simulink model "Appl_DrMotorAdjust_CtrlModel"  (R2018b)
settings: configuration reference "CodeConfig_10_ms" (kept outside this file)
undefined symbols (not defined in the file): CAL_HightMotorRunInterval_100ms, CAL_MotorDiffToStart_100ms, CAL_MotorStopTime_50ms, D_Relay_DownBackFault, D_Relay_UpFrontFault, D_ToleranceDistance, enSeatMoveCmd, FALSE, TRUE
libraries: DareLib x88, simulink x2
(part 3 of 3)

== stateflow chart Appl_DrMotorAdjust_CtrlModel/LogicCtrl/LocalAdjustCtrl/MotorAdjust/LengthMotorRun/MotorAdjust ==
  note: 此处取霍尔值越往下越大约往后越大
  state Init_Interval
    en:
    H_SeatMoveCmd = enSeatMoveCmd.EN_NULL;
    HMotorRunIntervalTime = 1;
    DownBackFlag = 0;
    UpFrontFlag = 0;
    Testvalue = 1;
    du:
    ex:
    HMotorRunIntervalTime = 0;
    Init_Interval -> (junction 11) [order 1]
    (junction 11) -> (junction 13) [order 1] : /*纵向电机调间隔时间*/
        | [HMotorRunIntervalTime < CAL_HightMotorRunInterval_100ms]
    (junction 11) -> (junction 17) [order 2]
    (junction 13) -> (junction 15) : {HMotorRunIntervalTime ++;}
    (junction 15) -> (junction 17)
    (junction 17) -> (junction 30) : {DownBackFlag = 0;
        | UpFrontFlag = 0;}
    (junction 30) -> (junction 32) [order 1] : /*纵向自动调节有效*/
        | [0 != SeatHeightPosiReq]
    (junction 32) -> (junction 43) [order 1] : /*纵向误差判断目前定义为5霍尔数值*/
        | [enSeatMoveCmd.EN_UP_FORWARD != LengthSoftStopFault ...
        | && SeatHeightPosiReq > DrAdj_InCurrentHallCnt ...
        | && D_ToleranceDistance < (SeatHeightPosiReq - DrAdj_InCurrentHallCnt)]
    (junction 30) -> (junction 39) [order 2] : { HeightAutoRunFlag = EN_SEAT_INVALID;}
    (junction 32) -> (junction 34) [order 2]
    (junction 43) -> (junction 45) : {UpFrontFlag = 1;}
    (junction 34) -> (junction 47) [order 1] : /* 不在软止点 且超误差范围 */
        | [enSeatMoveCmd.EN_DN_BACKWARD != LengthSoftStopFault ...
        | && SeatHeightPosiReq < DrAdj_InCurrentHallCnt ...
        | && D_ToleranceDistance < (DrAdj_InCurrentHallCnt - SeatHeightPosiReq)]
    (junction 34) -> (junction 52) [order 2] : /*纵向误差范围内，反馈成功*/
        | {HeightAutoRunFlag = EN_SEAT_SUCCESS;
        | H_MotorRunType = EN_AutoAdjust_FUSuccess_Stop;}
    (junction 47) -> (junction 49) : {DownBackFlag = 1;}
    (junction 52) -> (junction 39)
    (junction 49) -> (junction 52)
    (junction 45) -> (junction 49)
    (junction 39) -> (junction 57)
    (junction 57) -> (junction 134)
    (junction 134) -> (junction 135) [order 1] : /* 调用位置有变化 则先清状态 */
        | [hasChanged(SeatHeightPosiReq)]
    (junction 134) -> (junction 133) [order 2]
    (junction 135) -> (junction 126) : {HeightAutoRunFlag = EN_SEAT_INVALID;}
    (junction 126) -> (junction 133)
    (junction 133) -> (junction 128)
  state H_MotorUpFrontRun
    en:
    H_SeatMoveCmd  = EN_UP_FORWARD
    Testvalue = 2;
    (default) -> (junction 64)
    H_MotorUpFrontRun -> (junction 64) [order 1]
    (junction 64) -> (junction 67) [order 1] : /*自动调节*/
        | [EN_AutoAdjust_FU == H_MotorRunType]
    (junction 64) -> (junction 71) [order 2] : {HeightAutoRunFlag = EN_SEAT_INVALID;}
    (junction 67) -> (junction 69) : {HeightAutoRunFlag = EN_SEAT_RUNNING;}
    (junction 69) -> (junction 71)
    (junction 71) -> (junction 74)
  state H_MotorDownBackRun
    en:
    H_SeatMoveCmd  = EN_DN_BACKWARD;
    Testvalue = 3;
    (default) -> (junction 87)
    H_MotorDownBackRun -> (junction 87) [order 1]
    (junction 87) -> (junction 81) [order 1] : /*纵向自动调节*/
        | [EN_AutoAdjust_BK == H_MotorRunType]
    (junction 87) -> (junction 84) [order 2] : {HeightAutoRunFlag = EN_SEAT_INVALID;}
    (junction 81) -> (junction 77) : {HeightAutoRunFlag = EN_SEAT_RUNNING;}
    (junction 77) -> (junction 84)
    (junction 84) -> (junction 89)
  (default) -> Init_Interval
  Init_Interval -> H_MotorUpFrontRun [order 4] : /*纵向继电器下后粘连故障 == 有效 间隔时间大于100ms*/
      | [Relay_DownBackFault ==  Relay_FaultSts...
      | && CAL_HightMotorRunInterval_100ms <= HMotorRunIntervalTime ]
      | /H_MotorRunType = EN_DnBkRelayAdhesion_FU;
  Init_Interval -> H_MotorDownBackRun [order 1] : /*纵向继电器上前粘连故障 == 有效*/
      | [Relay_UpFrontFault == Relay_FaultSts ...
      | && CAL_HightMotorRunInterval_100ms <= HMotorRunIntervalTime ]
      | /H_MotorRunType = EN_DnFURelayAdhesion_BK;
  H_MotorUpFrontRun -> Init_Interval [order 3] : /*纵向继电器下后粘连故障 != 有效*/
      | [Relay_DownBackFault != Relay_FaultSts...
      | && EN_DnBkRelayAdhesion_FU == H_MotorRunType]
      | /H_MotorRunType = EN_DnBkRelayAdhesion_FU_Stop;
  H_MotorDownBackRun -> Init_Interval [order 9] : /*纵向继电器上前粘连故障 ！= 有效*/
      | [Relay_UpFrontFault != Relay_FaultSts  ...
      | && EN_DnFURelayAdhesion_BK == H_MotorRunType]
      | /H_MotorRunType = EN_DnFURelayAdhesion_BK_Stop;
  Init_Interval -> H_MotorUpFrontRun [order 3] : /*纵向手动调节*/
      | [EN_UP_FORWARD == HeightManualAdjSw ...
      | && FALSE == LengthLockFault  ...
      | && FALSE == LengthHallFault ...
      | && FALSE == TimeoutFlag ...
      | && CAL_HightMotorRunInterval_100ms <= HMotorRunIntervalTime]
      | /H_MotorRunType = EN_ManualAdjust_FU;
  Init_Interval -> H_MotorDownBackRun [order 6] : /*纵向手动调节有效*/
      | [EN_DN_BACKWARD == HeightManualAdjSw ...
      | && FALSE == LengthLockFault   ...
      | && FALSE == LengthHallFault...
      | && FALSE == TimeoutFlag ...
      | && CAL_HightMotorRunInterval_100ms <= HMotorRunIntervalTime]
      | /H_MotorRunType = EN_ManualAdjust_BK;
  H_MotorUpFrontRun -> Init_Interval [order 5] : /*纵向手动调节无效*/
      | [(EN_UP_FORWARD != HeightManualAdjSw) ...
      | && EN_ManualAdjust_FU == H_MotorRunType]
      | /H_MotorRunType = EN_ManualAdjust_FU_Stop;
  H_MotorDownBackRun -> Init_Interval [order 7] : /*纵向手动调节无效*/
      | [(EN_DN_BACKWARD != HeightManualAdjSw) ...
      | && EN_ManualAdjust_BK == H_MotorRunType]
      | /H_MotorRunType = EN_ManualAdjust_BK_Stop;
  Init_Interval -> H_MotorUpFrontRun [order 5] : /*纵向自动调节有效且不在误差范围内*/
      | [0 != SeatHeightPosiReq ...
      | && FALSE == LengthLockFault ...
      | && HeightAutoRunFlag == EN_SEAT_INVALID ...
      | && UpFrontFlag == 1 ...
      | && CAL_HightMotorRunInterval_100ms <= HMotorRunIntervalTime]
      | /H_MotorRunType = EN_AutoAdjust_FU;
  Init_Interval -> H_MotorDownBackRun [order 2] : /*纵向自动调节有效且不在误差范围内*/
      | [0 != SeatHeightPosiReq ...
      | && FALSE == LengthLockFault ...
      | && HeightAutoRunFlag == EN_SEAT_INVALID ...
      | && DownBackFlag == 1 ...
      | && CAL_HightMotorRunInterval_100ms <= HMotorRunIntervalTime]
      | /H_MotorRunType = EN_AutoAdjust_BK;
  H_MotorDownBackRun -> Init_Interval [order 3] : /*纵向自动调节无效 设置电机运行类型BK停止 自动运行标志位失败*/
      | [0 == SeatHeightPosiReq ...
      | && EN_AutoAdjust_BK == H_MotorRunType]
      | /H_MotorRunType = EN_AutoAdjust_BK_Stop;
      | HeightAutoRunFlag =EN_SEAT_FAIL;
  H_MotorUpFrontRun -> Init_Interval [order 6] : /*纵向自动调节无效 设置电机运行类型FU停止 自动运行标志位失败*/
      | [0 == SeatHeightPosiReq ...
      | && EN_AutoAdjust_FU == H_MotorRunType]
      | /H_MotorRunType = EN_AutoAdjust_FU_Stop;
      | HeightAutoRunFlag =EN_SEAT_FAIL
  H_MotorUpFrontRun -> Init_Interval [order 7] : /*纵向自动调节成功 设置电机运行类型FU成功停止 自动运行标志位成功*/
      | [EN_AutoAdjust_FU == H_MotorRunType ...
      | && D_ToleranceDistance >= abs(SeatHeightPosiReq -  DrAdj_InCurrentHallCnt)]
      | /HeightAutoRunFlag = EN_SEAT_SUCCESS;
      | H_MotorRunType = EN_AutoAdjust_FUSuccess_Stop;
  H_MotorDownBackRun -> Init_Interval [order 4] : /*自动调节成功 设置电机运行类型成功停止 自动运行标志位成功*/
      | [EN_AutoAdjust_BK == H_MotorRunType ...
      | && D_ToleranceDistance >= abs(DrAdj_InCurrentHallCnt  - SeatHeightPosiReq)]
      | /HeightAutoRunFlag = EN_SEAT_SUCCESS;
      | H_MotorRunType = EN_AutoAdjust_BKSuccess_Stop;
  H_MotorUpFrontRun -> Init_Interval [order 9] : /*纵向超时停止-非继电器粘连的驱动*/
      | [TRUE == TimeoutFlag ...
      | && Relay_DownBackFault !=  Relay_FaultSts]
      | /H_MotorRunType = EN_AutoAdjust_FUSuccess_Stop;
      | HeightAutoRunFlag =EN_SEAT_FAIL;
  H_MotorDownBackRun -> Init_Interval [order 8] : /*纵向超时停止-非继电器粘连的驱动*/
      | [TRUE == TimeoutFlag ...
      | && Relay_UpFrontFault != Relay_FaultSts]
      | /H_MotorRunType = EN_AutoAdjust_BKSuccess_Stop;
      | HeightAutoRunFlag =EN_SEAT_FAIL;
  H_MotorUpFrontRun -> Init_Interval [order 4] : /* 纵向向前到达止点，存在堵转故障，反馈成功 */
      | [/*FALSE == Relay_FaultSts &&*/ TRUE == LengthLockFault]
      | /H_MotorRunType = enSeatHightMotorRunsts.EN_UpFn_Lock_Stop;
      | HeightAutoRunFlag =EN_SEAT_SUCCESS;
  H_MotorDownBackRun -> Init_Interval [order 6] : /* 纵向向后到达止点，存在堵转故障，反馈成功 */
      | [/*FALSE == Relay_FaultSts &&*/ TRUE == LengthLockFault]/
      | H_MotorRunType = enSeatHightMotorRunsts.EN_DnBa_Lock_Stop;
      | HeightAutoRunFlag =EN_SEAT_SUCCESS;
  H_MotorUpFrontRun -> Init_Interval [order 10] : /* 纵向存在霍尔故障 */
      | [/*FALSE == Relay_FaultSts && */TRUE == LengthHallFault]
      | /H_MotorRunType = enSeatHightMotorRunsts.EN_UpFn_Hall_Stop;
      | HeightAutoRunFlag =EN_SEAT_FAIL;
  H_MotorDownBackRun -> Init_Interval [order 10] : /* 存在霍尔故障 */
      | [/*FALSE == Relay_FaultSts &&*/ TRUE == LengthHallFault]
      | /H_MotorRunType = enSeatHightMotorRunsts.EN_DnBa_Hall_Stop;
      | HeightAutoRunFlag =EN_SEAT_FAIL;
  H_MotorUpFrontRun -> Init_Interval [order 11] : /* 纵向存在MOS故障 */
      | [enMosErrSts.enNULL != MosErrSts]
      | /H_MotorRunType = enSeatHightMotorRunsts.EN_DnBa_MovTypeChange + MosErrSts;
      | HeightAutoRunFlag =EN_SEAT_FAIL;
  H_MotorDownBackRun -> Init_Interval [order 11] : /* 存在MOS故障 */
      | [enMosErrSts.enNULL != MosErrSts]
      | /H_MotorRunType = enSeatHightMotorRunsts.EN_DnBa_MovTypeChange + MosErrSts;
      | HeightAutoRunFlag =EN_SEAT_FAIL;
  H_MotorDownBackRun -> Init_Interval [order 2] : /*自动调节-到达软止点停止 成功 */
      |  [EN_AutoAdjust_BK == H_MotorRunType ...
      | && enSeatMoveCmd.EN_DN_BACKWARD == LengthSoftStopFault]
      | /HeightAutoRunFlag = EN_SEAT_SUCCESS;
      | H_MotorRunType = EN_AutoAdjust_BKSuccess_Stop;
  H_MotorUpFrontRun -> Init_Interval [order 1] : /*自动调节-到达软止点停止 成功 */
      |  [EN_AutoAdjust_FU == H_MotorRunType ...
      | && enSeatMoveCmd.EN_UP_FORWARD == LengthSoftStopFault]
      | /HeightAutoRunFlag = EN_SEAT_SUCCESS;
      | H_MotorRunType = EN_AutoAdjust_FUSuccess_Stop;
  H_MotorDownBackRun -> Init_Interval [order 1] : /*纵向控制类型改变
      | 优先级需要设定为1*/
      | [hasChanged(MotorActType)...
      |  && enSeatMotorRunTye.EN_NULL != MotorActType]
      | /HeightAutoRunFlag = EN_SEAT_INVALID;
      | H_MotorRunType = EN_DnBa_MovTypeChange;
  H_MotorUpFrontRun -> Init_Interval [order 2] : /*纵向控制类型改变
      | 不能返回运动成功优先级需要设定为1*/
      | [hasChanged(MotorActType)...
      |  && enSeatMotorRunTye.EN_NULL != MotorActType]
      | /HeightAutoRunFlag = EN_SEAT_INVALID;
      | H_MotorRunType = EN_UpFn_MovTypeChange
  H_MotorDownBackRun -> Init_Interval [order 5] : /* 不在软止点 且超过误差范围，需要向前驱动 */
      | [0 != SeatHeightPosiReq ...
      | && SeatHeightPosiReq > DrAdj_InCurrentHallCnt]
      | /HeightAutoRunFlag = EN_SEAT_INVALID;
      | H_MotorRunType = EN_AutoAdjust_BK_Stop;
  H_MotorUpFrontRun -> Init_Interval [order 8] : /* 不在软止点 且超过误差范围，需要向后驱动 */
      | [0 != SeatHeightPosiReq ...
      | && SeatHeightPosiReq < DrAdj_InCurrentHallCnt]
      | /HeightAutoRunFlag = EN_SEAT_INVALID;
      | H_MotorRunType = EN_AutoAdjust_FU_Stop;
  data: TimeoutFlag input; DrAdj_InCurrentHallCnt input; Relay_FaultSts input; SeatHeightPosiReq input; HeightManualAdjSw input; H_SeatMoveCmd output Enum: enSeatMoveCmd; H_MotorRunType output Enum: enSeatHightMotorRunsts; CAL_HightMotorRunInterval_100ms input; DownBackFlag local uint8; UpFrontFlag local uint8; HeightAutoRunFlag output Enum: enSeatAutoRunSts; TRUE input; HMotorRunIntervalTime local uint8 =10; Relay_DownBackFault input; Relay_UpFrontFault input; LengthHallFault input; LengthLockFault input; FALSE parameter; LengthSoftStopFault input; MotorActType input; D_ToleranceDistance input; Testvalue output uint8; MosErrSts input Enum: enMosErrSts

== stateflow chart Appl_DrMotorAdjust_CtrlModel/LogicCtrl/LocalAdjustCtrl/MotorAdjust/BackMotorRun/MotorAdjust ==
  note: 此处取霍尔值越往下越大约往后越大
  state Init_Interval
    en:
    H_SeatMoveCmd = enSeatMoveCmd.EN_NULL;
    HMotorRunIntervalTime = 1;
    DownBackFlag = 0;
    UpFrontFlag = 0;
    Testvalue = 1;
    du:
    ex:
    HMotorRunIntervalTime = 0;
    Init_Interval -> (junction 11) [order 1]
    (junction 11) -> (junction 13) [order 1] : /*靠背电机调间隔时间*/
        | [HMotorRunIntervalTime < CAL_HightMotorRunInterval_100ms]
    (junction 11) -> (junction 17) [order 2]
    (junction 13) -> (junction 15) : {HMotorRunIntervalTime ++;}
    (junction 15) -> (junction 17)
    (junction 17) -> (junction 30) : {DownBackFlag = 0;
        | UpFrontFlag = 0;}
    (junction 30) -> (junction 32) [order 1] : /*靠背自动调节有效*/
        | [0 != SeatHeightPosiReq]
    (junction 32) -> (junction 43) [order 1] : /*靠背误差判断目前定义为5霍尔数值*/
        | [enSeatMoveCmd.EN_UP_FORWARD != LengthSoftStopFault ...
        | && SeatHeightPosiReq > DrAdj_InCurrentHallCnt ...
        | && D_ToleranceDistance < (SeatHeightPosiReq - DrAdj_InCurrentHallCnt)]
    (junction 30) -> (junction 39) [order 2] : { HeightAutoRunFlag = EN_SEAT_INVALID;}
    (junction 32) -> (junction 34) [order 2]
    (junction 43) -> (junction 45) : {UpFrontFlag = 1;}
    (junction 34) -> (junction 47) [order 1] : /* 不在软止点 且超误差范围 */
        | [enSeatMoveCmd.EN_DN_BACKWARD != LengthSoftStopFault ...
        | && SeatHeightPosiReq < DrAdj_InCurrentHallCnt ...
        | && D_ToleranceDistance < (DrAdj_InCurrentHallCnt - SeatHeightPosiReq)]
    (junction 34) -> (junction 52) [order 2] : /*靠背误差范围内，反馈成功*/
        | {HeightAutoRunFlag = EN_SEAT_SUCCESS;
        | H_MotorRunType = EN_AutoAdjust_FUSuccess_Stop;}
    (junction 47) -> (junction 49) : {DownBackFlag = 1;}
    (junction 52) -> (junction 39)
    (junction 49) -> (junction 52)
    (junction 45) -> (junction 49)
    (junction 39) -> (junction 57)
    (junction 57) -> (junction 134)
    (junction 134) -> (junction 135) [order 1] : /* 调用位置有变化 则先清状态 */
        | [hasChanged(SeatHeightPosiReq)]
    (junction 134) -> (junction 133) [order 2]
    (junction 135) -> (junction 126) : {HeightAutoRunFlag = EN_SEAT_INVALID;}
    (junction 126) -> (junction 133)
    (junction 133) -> (junction 128)
  state H_MotorUpFrontRun
    en:
    H_SeatMoveCmd  = EN_UP_FORWARD
    Testvalue = 2;
    (default) -> (junction 64)
    H_MotorUpFrontRun -> (junction 64) [order 1]
    (junction 64) -> (junction 67) [order 1] : /*自动调节*/
        | [EN_AutoAdjust_FU == H_MotorRunType]
    (junction 64) -> (junction 71) [order 2] : {HeightAutoRunFlag = EN_SEAT_INVALID;}
    (junction 67) -> (junction 69) : {HeightAutoRunFlag = EN_SEAT_RUNNING;}
    (junction 69) -> (junction 71)
    (junction 71) -> (junction 74)
  state H_MotorDownBackRun
    en:
    H_SeatMoveCmd  = EN_DN_BACKWARD;
    Testvalue = 3;
    (default) -> (junction 87)
    H_MotorDownBackRun -> (junction 87) [order 1]
    (junction 87) -> (junction 81) [order 1] : /*靠背自动调节*/
        | [EN_AutoAdjust_BK == H_MotorRunType]
    (junction 87) -> (junction 84) [order 2] : {HeightAutoRunFlag = EN_SEAT_INVALID;}
    (junction 81) -> (junction 77) : {HeightAutoRunFlag = EN_SEAT_RUNNING;}
    (junction 77) -> (junction 84)
    (junction 84) -> (junction 89)
  (default) -> Init_Interval
  Init_Interval -> H_MotorUpFrontRun [order 4] : /*靠背继电器下后粘连故障 == 有效 间隔时间大于100ms*/
      | [Relay_DownBackFault ==  Relay_FaultSts...
      | && CAL_HightMotorRunInterval_100ms <= HMotorRunIntervalTime ]
      | /H_MotorRunType = EN_DnBkRelayAdhesion_FU;
  Init_Interval -> H_MotorDownBackRun [order 1] : /*靠背继电器上前粘连故障 == 有效*/
      | [Relay_UpFrontFault == Relay_FaultSts ...
      | && CAL_HightMotorRunInterval_100ms <= HMotorRunIntervalTime ]
      | /H_MotorRunType = EN_DnFURelayAdhesion_BK;
  H_MotorUpFrontRun -> Init_Interval [order 3] : /*靠背继电器下后粘连故障 != 有效*/
      | [Relay_DownBackFault != Relay_FaultSts...
      | && EN_DnBkRelayAdhesion_FU == H_MotorRunType]
      | /H_MotorRunType = EN_DnBkRelayAdhesion_FU_Stop;
  H_MotorDownBackRun -> Init_Interval [order 9] : /*靠背继电器上前粘连故障 ！= 有效*/
      | [Relay_UpFrontFault != Relay_FaultSts  ...
      | && EN_DnFURelayAdhesion_BK == H_MotorRunType]
      | /H_MotorRunType = EN_DnFURelayAdhesion_BK_Stop;
  Init_Interval -> H_MotorUpFrontRun [order 3] : /*靠背手动调节*/
      | [EN_UP_FORWARD == HeightManualAdjSw ...
      | && FALSE == LengthLockFault  ...
      | && FALSE == LengthHallFault ...
      | && FALSE == TimeoutFlag ...
      | && CAL_HightMotorRunInterval_100ms <= HMotorRunIntervalTime]
      | /H_MotorRunType = EN_ManualAdjust_FU;
  Init_Interval -> H_MotorDownBackRun [order 6] : /*靠背手动调节有效*/
      | [EN_DN_BACKWARD == HeightManualAdjSw ...
      | && FALSE == LengthLockFault   ...
      | && FALSE == LengthHallFault...
      | && FALSE == TimeoutFlag ...
      | && CAL_HightMotorRunInterval_100ms <= HMotorRunIntervalTime]
      | /H_MotorRunType = EN_ManualAdjust_BK;
  H_MotorUpFrontRun -> Init_Interval [order 5] : /*靠背手动调节无效*/
      | [(EN_UP_FORWARD != HeightManualAdjSw) ...
      | && EN_ManualAdjust_FU == H_MotorRunType]
      | /H_MotorRunType = EN_ManualAdjust_FU_Stop;
  H_MotorDownBackRun -> Init_Interval [order 7] : /*靠背手动调节无效*/
      | [(EN_DN_BACKWARD != HeightManualAdjSw) ...
      | && EN_ManualAdjust_BK == H_MotorRunType]
      | /H_MotorRunType = EN_ManualAdjust_BK_Stop;
  Init_Interval -> H_MotorUpFrontRun [order 5] : /*靠背自动调节有效且不在误差范围内*/
      | [0 != SeatHeightPosiReq ...
      | && FALSE == LengthLockFault ...
      | && HeightAutoRunFlag == EN_SEAT_INVALID ...
      | && UpFrontFlag == 1 ...
      | && CAL_HightMotorRunInterval_100ms <= HMotorRunIntervalTime]
      | /H_MotorRunType = EN_AutoAdjust_FU;
  Init_Interval -> H_MotorDownBackRun [order 2] : /*靠背自动调节有效且不在误差范围内*/
      | [0 != SeatHeightPosiReq ...
      | && FALSE == LengthLockFault ...
      | && HeightAutoRunFlag == EN_SEAT_INVALID ...
      | && DownBackFlag == 1 ...
      | && CAL_HightMotorRunInterval_100ms <= HMotorRunIntervalTime]
      | /H_MotorRunType = EN_AutoAdjust_BK;
  H_MotorDownBackRun -> Init_Interval [order 3] : /*靠背自动调节无效 设置电机运行类型BK停止 自动运行标志位失败*/
      | [0 == SeatHeightPosiReq ...
      | && EN_AutoAdjust_BK == H_MotorRunType]
      | /H_MotorRunType = EN_AutoAdjust_BK_Stop;
      | HeightAutoRunFlag =EN_SEAT_FAIL;
  H_MotorUpFrontRun -> Init_Interval [order 6] : /*靠背自动调节无效 设置电机运行类型FU停止 自动运行标志位失败*/
      | [0 == SeatHeightPosiReq ...
      | && EN_AutoAdjust_FU == H_MotorRunType]
      | /H_MotorRunType = EN_AutoAdjust_FU_Stop;
      | HeightAutoRunFlag =EN_SEAT_FAIL
  H_MotorUpFrontRun -> Init_Interval [order 7] : /*靠背自动调节成功 设置电机运行类型FU成功停止 自动运行标志位成功*/
      | [EN_AutoAdjust_FU == H_MotorRunType ...
      | && D_ToleranceDistance >= abs(SeatHeightPosiReq -  DrAdj_InCurrentHallCnt)]
      | /HeightAutoRunFlag = EN_SEAT_SUCCESS;
      | H_MotorRunType = EN_AutoAdjust_FUSuccess_Stop;
  H_MotorDownBackRun -> Init_Interval [order 4] : /*自动调节成功 设置电机运行类型成功停止 自动运行标志位成功*/
      | [EN_AutoAdjust_BK == H_MotorRunType ...
      | && D_ToleranceDistance >= abs(DrAdj_InCurrentHallCnt  - SeatHeightPosiReq)]
      | /HeightAutoRunFlag = EN_SEAT_SUCCESS;
      | H_MotorRunType = EN_AutoAdjust_BKSuccess_Stop;
  H_MotorUpFrontRun -> Init_Interval [order 9] : /*靠背超时停止-非继电器粘连的驱动*/
      | [TRUE == TimeoutFlag ...
      | && Relay_DownBackFault !=  Relay_FaultSts]
      | /H_MotorRunType = EN_AutoAdjust_FUSuccess_Stop;
      | HeightAutoRunFlag =EN_SEAT_FAIL;
  H_MotorDownBackRun -> Init_Interval [order 8] : /*靠背超时停止-非继电器粘连的驱动*/
      | [TRUE == TimeoutFlag ...
      | && Relay_UpFrontFault != Relay_FaultSts]
      | /H_MotorRunType = EN_AutoAdjust_BKSuccess_Stop;
      | HeightAutoRunFlag =EN_SEAT_FAIL;
  H_MotorUpFrontRun -> Init_Interval [order 4] : /* 靠背向前到达止点，存在堵转故障，反馈成功 */
      | [/*FALSE == Relay_FaultSts &&*/ TRUE == LengthLockFault]
      | /H_MotorRunType = enSeatHightMotorRunsts.EN_UpFn_Lock_Stop;
      | HeightAutoRunFlag =EN_SEAT_SUCCESS;
  H_MotorDownBackRun -> Init_Interval [order 6] : /* 靠背向后到达止点，存在堵转故障，反馈成功 */
      | [/*FALSE == Relay_FaultSts &&*/ TRUE == LengthLockFault]/
      | H_MotorRunType = enSeatHightMotorRunsts.EN_DnBa_Lock_Stop;
      | HeightAutoRunFlag =EN_SEAT_SUCCESS;
  H_MotorDownBackRun -> Init_Interval [order 10] : /* 存在霍尔故障 */
      | [/*FALSE == Relay_FaultSts &&*/ TRUE == LengthHallFault]
      | /H_MotorRunType = enSeatHightMotorRunsts.EN_DnBa_Hall_Stop;
      | HeightAutoRunFlag =EN_SEAT_FAIL;
  H_MotorUpFrontRun -> Init_Interval [order 10] : /* 靠背存在霍尔故障 */
      | [/*FALSE == Relay_FaultSts && */TRUE == LengthHallFault]
      | /H_MotorRunType = enSeatHightMotorRunsts.EN_UpFn_Hall_Stop;
      | HeightAutoRunFlag =EN_SEAT_FAIL;
  H_MotorDownBackRun -> Init_Interval [order 11] : /* 存在MOS故障 */
      | [enMosErrSts.enNULL != MosErrSts]
      | /H_MotorRunType = enSeatHightMotorRunsts.EN_DnBa_MovTypeChange + MosErrSts;
      | HeightAutoRunFlag =EN_SEAT_FAIL;
  H_MotorUpFrontRun -> Init_Interval [order 11] : /* 靠背存在MOS故障 */
      | [enMosErrSts.enNULL != MosErrSts]
      | /H_MotorRunType = enSeatHightMotorRunsts.EN_DnBa_MovTypeChange + MosErrSts;
      | HeightAutoRunFlag =EN_SEAT_FAIL;
  H_MotorDownBackRun -> Init_Interval [order 2] : /*自动调节-到达软止点停止 成功 */
      |  [EN_AutoAdjust_BK == H_MotorRunType ...
      | && enSeatMoveCmd.EN_DN_BACKWARD == LengthSoftStopFault]
      | /HeightAutoRunFlag = EN_SEAT_SUCCESS;
      | H_MotorRunType = EN_AutoAdjust_BKSuccess_Stop;
  H_MotorUpFrontRun -> Init_Interval [order 1] : /*自动调节-到达软止点停止 成功 */
      |  [EN_AutoAdjust_FU == H_MotorRunType ...
      | && enSeatMoveCmd.EN_UP_FORWARD == LengthSoftStopFault]
      | /HeightAutoRunFlag = EN_SEAT_SUCCESS;
      | H_MotorRunType = EN_AutoAdjust_FUSuccess_Stop;
  H_MotorDownBackRun -> Init_Interval [order 1] : /*靠背控制类型改变
      | 优先级需要设定为1*/
      | [hasChanged(MotorActType)...
      |  && enSeatMotorRunTye.EN_NULL != MotorActType]
      | /HeightAutoRunFlag = EN_SEAT_INVALID;
      | H_MotorRunType = EN_DnBa_MovTypeChange;
  H_MotorUpFrontRun -> Init_Interval [order 2] : /*靠背控制类型改变
      | 不能返回运动成功优先级需要设定为1*/
      | [hasChanged(MotorActType)...
      |  && enSeatMotorRunTye.EN_NULL != MotorActType]
      | /HeightAutoRunFlag = EN_SEAT_INVALID;
      | H_MotorRunType = EN_UpFn_MovTypeChange
  H_MotorDownBackRun -> Init_Interval [order 5] : /* 不在软止点 且超过误差范围，需要向前驱动 */
      | [0 != SeatHeightPosiReq ...
      | && SeatHeightPosiReq > DrAdj_InCurrentHallCnt]
      | /HeightAutoRunFlag = EN_SEAT_INVALID;
      | H_MotorRunType = EN_AutoAdjust_BK_Stop;
  H_MotorUpFrontRun -> Init_Interval [order 8] : /* 不在软止点 且超过误差范围，需要向后驱动 */
      | [0 != SeatHeightPosiReq ...
      | && SeatHeightPosiReq < DrAdj_InCurrentHallCnt]
      | /HeightAutoRunFlag = EN_SEAT_INVALID;
      | H_MotorRunType = EN_AutoAdjust_FU_Stop;
  data: TimeoutFlag input; DrAdj_InCurrentHallCnt input; Relay_FaultSts input; SeatHeightPosiReq input; HeightManualAdjSw input; H_SeatMoveCmd output Enum: enSeatMoveCmd; H_MotorRunType output Enum: enSeatHightMotorRunsts; CAL_HightMotorRunInterval_100ms input; DownBackFlag local uint8; UpFrontFlag local uint8; HeightAutoRunFlag output Enum: enSeatAutoRunSts; TRUE input; HMotorRunIntervalTime local uint8 =10; Relay_DownBackFault input; Relay_UpFrontFault input; LengthHallFault input; LengthLockFault input; FALSE parameter; LengthSoftStopFault input; MotorActType input; D_ToleranceDistance input; Testvalue output uint8; MosErrSts input Enum: enMosErrSts

== stateflow chart Appl_DrMotorAdjust_CtrlModel/LogicCtrl/LocalAdjustCtrl/MotorAdjust/FrontMotorRun/MotorAdjust ==
  note: 此处取霍尔值越往下越大约往后越大
  state Init_Interval
    en:
    H_SeatMoveCmd = enSeatMoveCmd.EN_NULL;
    HMotorRunIntervalTime = 1;
    DownBackFlag = 0;
    UpFrontFlag = 0;
    Testvalue = 1;
    du:
    ex:
    HMotorRunIntervalTime = 0;
    Init_Interval -> (junction 11) [order 1]
    (junction 11) -> (junction 13) [order 1] : /*腿托电机调间隔时间*/
        | [HMotorRunIntervalTime < CAL_HightMotorRunInterval_100ms]
    (junction 11) -> (junction 17) [order 2]
    (junction 13) -> (junction 15) : {HMotorRunIntervalTime ++;}
    (junction 15) -> (junction 17)
    (junction 17) -> (junction 30) : {DownBackFlag = 0;
        | UpFrontFlag = 0;}
    (junction 30) -> (junction 32) [order 1] : /*腿托自动调节有效*/
        | [0 != SeatHeightPosiReq]
    (junction 32) -> (junction 43) [order 1] : /*腿托误差判断目前定义为5霍尔数值*/
        | [enSeatMoveCmd.EN_UP_FORWARD != LengthSoftStopFault ...
        | && SeatHeightPosiReq > DrAdj_InCurrentHallCnt ...
        | && D_ToleranceDistance < (SeatHeightPosiReq - DrAdj_InCurrentHallCnt)]
    (junction 30) -> (junction 39) [order 2] : { HeightAutoRunFlag = EN_SEAT_INVALID;}
    (junction 32) -> (junction 34) [order 2]
    (junction 43) -> (junction 45) : {UpFrontFlag = 1;}
    (junction 34) -> (junction 47) [order 1] : /* 不在软止点 且超误差范围 */
        | [enSeatMoveCmd.EN_DN_BACKWARD != LengthSoftStopFault ...
        | && SeatHeightPosiReq < DrAdj_InCurrentHallCnt ...
        | && D_ToleranceDistance < (DrAdj_InCurrentHallCnt - SeatHeightPosiReq)]
    (junction 34) -> (junction 52) [order 2] : /*腿托误差范围内，反馈成功*/
        | {HeightAutoRunFlag = EN_SEAT_SUCCESS;
        | H_MotorRunType = EN_AutoAdjust_FUSuccess_Stop;}
    (junction 47) -> (junction 49) : {DownBackFlag = 1;}
    (junction 52) -> (junction 39)
    (junction 49) -> (junction 52)
    (junction 45) -> (junction 49)
    (junction 39) -> (junction 57)
    (junction 57) -> (junction 134)
    (junction 134) -> (junction 135) [order 1] : /* 调用位置有变化 则先清状态 */
        | [hasChanged(SeatHeightPosiReq)]
    (junction 134) -> (junction 133) [order 2]
    (junction 135) -> (junction 126) : {HeightAutoRunFlag = EN_SEAT_INVALID;}
    (junction 126) -> (junction 133)
    (junction 133) -> (junction 128)
  state H_MotorUpFrontRun
    en:
    H_SeatMoveCmd  = EN_UP_FORWARD
    Testvalue = 2;
    (default) -> (junction 64)
    H_MotorUpFrontRun -> (junction 64) [order 1]
    (junction 64) -> (junction 67) [order 1] : /*自动调节*/
        | [EN_AutoAdjust_FU == H_MotorRunType]
    (junction 64) -> (junction 71) [order 2] : {HeightAutoRunFlag = EN_SEAT_INVALID;}
    (junction 67) -> (junction 69) : {HeightAutoRunFlag = EN_SEAT_RUNNING;}
    (junction 69) -> (junction 71)
    (junction 71) -> (junction 74)
  state H_MotorDownBackRun
    en:
    H_SeatMoveCmd  = EN_DN_BACKWARD;
    Testvalue = 3;
    (default) -> (junction 87)
    H_MotorDownBackRun -> (junction 87) [order 1]
    (junction 87) -> (junction 81) [order 1] : /*腿托自动调节*/
        | [EN_AutoAdjust_BK == H_MotorRunType]
    (junction 87) -> (junction 84) [order 2] : {HeightAutoRunFlag = EN_SEAT_INVALID;}
    (junction 81) -> (junction 77) : {HeightAutoRunFlag = EN_SEAT_RUNNING;}
    (junction 77) -> (junction 84)
    (junction 84) -> (junction 89)
  (default) -> Init_Interval
  Init_Interval -> H_MotorUpFrontRun [order 4] : /*腿托继电器下后粘连故障 == 有效 间隔时间大于100ms*/
      | [Relay_DownBackFault ==  Relay_FaultSts...
      | && CAL_HightMotorRunInterval_100ms <= HMotorRunIntervalTime ]
      | /H_MotorRunType = EN_DnBkRelayAdhesion_FU;
  Init_Interval -> H_MotorDownBackRun [order 1] : /*腿托继电器上前粘连故障 == 有效*/
      | [Relay_UpFrontFault == Relay_FaultSts ...
      | && CAL_HightMotorRunInterval_100ms <= HMotorRunIntervalTime ]
      | /H_MotorRunType = EN_DnFURelayAdhesion_BK;
  H_MotorUpFrontRun -> Init_Interval [order 3] : /*腿托继电器下后粘连故障 != 有效*/
      | [Relay_DownBackFault != Relay_FaultSts...
      | && EN_DnBkRelayAdhesion_FU == H_MotorRunType]
      | /H_MotorRunType = EN_DnBkRelayAdhesion_FU_Stop;
  H_MotorDownBackRun -> Init_Interval [order 9] : /*腿托继电器上前粘连故障 ！= 有效*/
      | [Relay_UpFrontFault != Relay_FaultSts  ...
      | && EN_DnFURelayAdhesion_BK == H_MotorRunType]
      | /H_MotorRunType = EN_DnFURelayAdhesion_BK_Stop;
  Init_Interval -> H_MotorUpFrontRun [order 3] : /*腿托手动调节*/
      | [EN_UP_FORWARD == HeightManualAdjSw ...
      | && FALSE == LengthLockFault  ...
      | && FALSE == LengthHallFault ...
      | && FALSE == TimeoutFlag ...
      | && CAL_HightMotorRunInterval_100ms <= HMotorRunIntervalTime]
      | /H_MotorRunType = EN_ManualAdjust_FU;
  Init_Interval -> H_MotorDownBackRun [order 6] : /*腿托手动调节有效*/
      | [EN_DN_BACKWARD == HeightManualAdjSw ...
      | && FALSE == LengthLockFault   ...
      | && FALSE == LengthHallFault...
      | && FALSE == TimeoutFlag ...
      | && CAL_HightMotorRunInterval_100ms <= HMotorRunIntervalTime]
      | /H_MotorRunType = EN_ManualAdjust_BK;
  H_MotorUpFrontRun -> Init_Interval [order 5] : /*腿托手动调节无效*/
      | [(EN_UP_FORWARD != HeightManualAdjSw) ...
      | && EN_ManualAdjust_FU == H_MotorRunType]
      | /H_MotorRunType = EN_ManualAdjust_FU_Stop;
  H_MotorDownBackRun -> Init_Interval [order 7] : /*腿托手动调节无效*/
      | [(EN_DN_BACKWARD != HeightManualAdjSw) ...
      | && EN_ManualAdjust_BK == H_MotorRunType]
      | /H_MotorRunType = EN_ManualAdjust_BK_Stop;
  Init_Interval -> H_MotorUpFrontRun [order 5] : /*腿托自动调节有效且不在误差范围内*/
      | [0 != SeatHeightPosiReq ...
      | && FALSE == LengthLockFault ...
      | && HeightAutoRunFlag == EN_SEAT_INVALID ...
      | && UpFrontFlag == 1 ...
      | && CAL_HightMotorRunInterval_100ms <= HMotorRunIntervalTime]
      | /H_MotorRunType = EN_AutoAdjust_FU;
  Init_Interval -> H_MotorDownBackRun [order 2] : /*腿托自动调节有效且不在误差范围内*/
      | [0 != SeatHeightPosiReq ...
      | && FALSE == LengthLockFault ...
      | && HeightAutoRunFlag == EN_SEAT_INVALID ...
      | && DownBackFlag == 1 ...
      | && CAL_HightMotorRunInterval_100ms <= HMotorRunIntervalTime]
      | /H_MotorRunType = EN_AutoAdjust_BK;
  H_MotorDownBackRun -> Init_Interval [order 3] : /*腿托自动调节无效 设置电机运行类型BK停止 自动运行标志位失败*/
      | [0 == SeatHeightPosiReq ...
      | && EN_AutoAdjust_BK == H_MotorRunType]
      | /H_MotorRunType = EN_AutoAdjust_BK_Stop;
      | HeightAutoRunFlag =EN_SEAT_FAIL;
  H_MotorUpFrontRun -> Init_Interval [order 6] : /*腿托自动调节无效 设置电机运行类型FU停止 自动运行标志位失败*/
      | [0 == SeatHeightPosiReq ...
      | && EN_AutoAdjust_FU == H_MotorRunType]
      | /H_MotorRunType = EN_AutoAdjust_FU_Stop;
      | HeightAutoRunFlag =EN_SEAT_FAIL
  H_MotorUpFrontRun -> Init_Interval [order 7] : /*腿托自动调节成功 设置电机运行类型FU成功停止 自动运行标志位成功*/
      | [EN_AutoAdjust_FU == H_MotorRunType ...
      | && D_ToleranceDistance >= abs(SeatHeightPosiReq -  DrAdj_InCurrentHallCnt)]
      | /HeightAutoRunFlag = EN_SEAT_SUCCESS;
      | H_MotorRunType = EN_AutoAdjust_FUSuccess_Stop;
  H_MotorDownBackRun -> Init_Interval [order 4] : /*自动调节成功 设置电机运行类型成功停止 自动运行标志位成功*/
      | [EN_AutoAdjust_BK == H_MotorRunType ...
      | && D_ToleranceDistance >= abs(DrAdj_InCurrentHallCnt  - SeatHeightPosiReq)]
      | /HeightAutoRunFlag = EN_SEAT_SUCCESS;
      | H_MotorRunType = EN_AutoAdjust_BKSuccess_Stop;
  H_MotorUpFrontRun -> Init_Interval [order 9] : /*腿托超时停止-非继电器粘连的驱动*/
      | [TRUE == TimeoutFlag ...
      | && Relay_DownBackFault !=  Relay_FaultSts]
      | /H_MotorRunType = EN_AutoAdjust_FUSuccess_Stop;
      | HeightAutoRunFlag =EN_SEAT_FAIL;
  H_MotorDownBackRun -> Init_Interval [order 8] : /*腿托超时停止-非继电器粘连的驱动*/
      | [TRUE == TimeoutFlag ...
      | && Relay_UpFrontFault != Relay_FaultSts]
      | /H_MotorRunType = EN_AutoAdjust_BKSuccess_Stop;
      | HeightAutoRunFlag =EN_SEAT_FAIL;
  H_MotorUpFrontRun -> Init_Interval [order 4] : /* 腿托向前到达止点，存在堵转故障，反馈成功 */
      | [/*FALSE == Relay_FaultSts &&*/ TRUE == LengthLockFault]
      | /H_MotorRunType = enSeatHightMotorRunsts.EN_UpFn_Lock_Stop;
      | HeightAutoRunFlag =EN_SEAT_SUCCESS;
  H_MotorDownBackRun -> Init_Interval [order 6] : /* 腿托向后到达止点，存在堵转故障，反馈成功 */
      | [/*FALSE == Relay_FaultSts &&*/ TRUE == LengthLockFault]/
      | H_MotorRunType = enSeatHightMotorRunsts.EN_DnBa_Lock_Stop;
      | HeightAutoRunFlag =EN_SEAT_SUCCESS;
  H_MotorDownBackRun -> Init_Interval [order 10] : /* 存在霍尔故障 */
      | [/*FALSE == Relay_FaultSts &&*/ TRUE == LengthHallFault]
      | /H_MotorRunType = enSeatHightMotorRunsts.EN_DnBa_Hall_Stop;
      | HeightAutoRunFlag =EN_SEAT_FAIL;
  H_MotorUpFrontRun -> Init_Interval [order 10] : /* 腿托存在霍尔故障 */
      | [/*FALSE == Relay_FaultSts && */TRUE == LengthHallFault]
      | /H_MotorRunType = enSeatHightMotorRunsts.EN_UpFn_Hall_Stop;
      | HeightAutoRunFlag =EN_SEAT_FAIL;
  H_MotorDownBackRun -> Init_Interval [order 11] : /* 存在MOS故障 */
      | [enMosErrSts.enNULL != MosErrSts]
      | /H_MotorRunType = enSeatHightMotorRunsts.EN_DnBa_MovTypeChange + MosErrSts;
      | HeightAutoRunFlag =EN_SEAT_FAIL;
  H_MotorUpFrontRun -> Init_Interval [order 11] : /* 腿托存在MOS故障 */
      | [enMosErrSts.enNULL != MosErrSts]
      | /H_MotorRunType = enSeatHightMotorRunsts.EN_DnBa_MovTypeChange + MosErrSts;
      | HeightAutoRunFlag =EN_SEAT_FAIL;
  H_MotorDownBackRun -> Init_Interval [order 2] : /*自动调节-到达软止点停止 成功 */
      |  [EN_AutoAdjust_BK == H_MotorRunType ...
      | && enSeatMoveCmd.EN_DN_BACKWARD == LengthSoftStopFault]
      | /HeightAutoRunFlag = EN_SEAT_SUCCESS;
      | H_MotorRunType = EN_AutoAdjust_BKSuccess_Stop;
  H_MotorUpFrontRun -> Init_Interval [order 1] : /*自动调节-到达软止点停止 成功 */
      |  [EN_AutoAdjust_FU == H_MotorRunType ...
      | && enSeatMoveCmd.EN_UP_FORWARD == LengthSoftStopFault]
      | /HeightAutoRunFlag = EN_SEAT_SUCCESS;
      | H_MotorRunType = EN_AutoAdjust_FUSuccess_Stop;
  H_MotorDownBackRun -> Init_Interval [order 1] : /*腿托控制类型改变
      | 优先级需要设定为1*/
      | [hasChanged(MotorActType)...
      |  && enSeatMotorRunTye.EN_NULL != MotorActType]
      | /HeightAutoRunFlag = EN_SEAT_INVALID;
      | H_MotorRunType = EN_DnBa_MovTypeChange;
  H_MotorUpFrontRun -> Init_Interval [order 2] : /*腿托控制类型改变
      | 不能返回运动成功优先级需要设定为1*/
      | [hasChanged(MotorActType)...
      |  && enSeatMotorRunTye.EN_NULL != MotorActType]
      | /HeightAutoRunFlag = EN_SEAT_INVALID;
      | H_MotorRunType = EN_UpFn_MovTypeChange
  H_MotorDownBackRun -> Init_Interval [order 5] : /* 不在软止点 且超过误差范围，需要向前驱动 */
      | [0 != SeatHeightPosiReq ...
      | && SeatHeightPosiReq > DrAdj_InCurrentHallCnt]
      | /HeightAutoRunFlag = EN_SEAT_INVALID;
      | H_MotorRunType = EN_AutoAdjust_BK_Stop;
  H_MotorUpFrontRun -> Init_Interval [order 8] : /* 不在软止点 且超过误差范围，需要向后驱动 */
      | [0 != SeatHeightPosiReq ...
      | && SeatHeightPosiReq < DrAdj_InCurrentHallCnt]
      | /HeightAutoRunFlag = EN_SEAT_INVALID;
      | H_MotorRunType = EN_AutoAdjust_FU_Stop;
  data: TimeoutFlag input; DrAdj_InCurrentHallCnt input; Relay_FaultSts input; SeatHeightPosiReq input; HeightManualAdjSw input; H_SeatMoveCmd output Enum: enSeatMoveCmd; H_MotorRunType output Enum: enSeatHightMotorRunsts; CAL_HightMotorRunInterval_100ms input; DownBackFlag local uint8; UpFrontFlag local uint8; HeightAutoRunFlag output Enum: enSeatAutoRunSts; TRUE input; HMotorRunIntervalTime local uint8 =10; Relay_DownBackFault input; Relay_UpFrontFault input; LengthHallFault input; LengthLockFault input; FALSE parameter; LengthSoftStopFault input; MotorActType input; D_ToleranceDistance input; Testvalue output uint8; MosErrSts input Enum: enMosErrSts

== stateflow chart Appl_DrMotorAdjust_CtrlModel/LogicCtrl/LocalAdjustCtrl/FourMotorPriority/HeightDelay ==
  state Height
    (default) -> (junction 7)
    Height -> (junction 7)
    (junction 7) -> (junction 10) [order 1] : [hasChangedTo(Can_MotorCtrl,0)]
    (junction 7) -> (junction 14) [order 2]
    (junction 10) -> (junction 12) : {StartFlag = TRUE;}
    (junction 12) -> (junction 14)
    (junction 14) -> (junction 17)
    (junction 17) -> (junction 19) [order 1] : /*延时50ms更新接口命令，避免Hall计数错误*/
        | [TRUE == StartFlag]
    (junction 17) -> (junction 28) [order 2] : {Command = Can_MotorCtrl;}
    (junction 19) -> (junction 21)
    (junction 21) -> (junction 31) [order 1] : [CAL_MotorStopTime_50ms > WaitTimer]
    (junction 21) -> (junction 35) [order 2] : {StartFlag = FALSE;
        | WaitTimer = 0;
        | Command = Can_MotorCtrl;}
    (junction 31) -> (junction 33) : {WaitTimer ++;}
    (junction 35) -> (junction 28)
    (junction 33) -> (junction 35)
    (junction 28) -> (junction 39)
  (default) -> Height
  data: Can_MotorCtrl input uint8; StartFlag local uint8; TRUE parameter; WaitTimer local uint8; CAL_MotorStopTime_50ms parameter; Command output uint8; FALSE parameter

== stateflow chart Appl_DrMotorAdjust_CtrlModel/LogicCtrl/LocalAdjustCtrl/FourMotorPriority/LengthDelay ==
  state Height
    (default) -> (junction 7)
    Height -> (junction 7)
    (junction 7) -> (junction 10) [order 1] : [hasChangedTo(Can_MotorCtrl,0)]
    (junction 7) -> (junction 14) [order 2]
    (junction 10) -> (junction 12) : {StartFlag = TRUE;}
    (junction 12) -> (junction 14)
    (junction 14) -> (junction 17)
    (junction 17) -> (junction 19) [order 1] : /*延时50ms更新接口命令，避免Hall计数错误*/
        | [TRUE == StartFlag]
    (junction 17) -> (junction 28) [order 2] : {Command = Can_MotorCtrl;}
    (junction 19) -> (junction 21)
    (junction 21) -> (junction 31) [order 1] : [CAL_MotorStopTime_50ms > WaitTimer]
    (junction 21) -> (junction 35) [order 2] : {StartFlag = FALSE;
        | WaitTimer = 0;
        | Command = Can_MotorCtrl;}
    (junction 31) -> (junction 33) : {WaitTimer ++;}
    (junction 35) -> (junction 28)
    (junction 33) -> (junction 35)
    (junction 28) -> (junction 39)
  (default) -> Height
  data: Can_MotorCtrl input uint8; StartFlag local uint8; TRUE parameter; WaitTimer local uint8; CAL_MotorStopTime_50ms parameter; Command output uint8; FALSE parameter

== stateflow chart Appl_DrMotorAdjust_CtrlModel/LogicCtrl/LocalAdjustCtrl/FourMotorPriority/BackDelay ==
  state Height
    (default) -> (junction 7)
    Height -> (junction 7)
    (junction 7) -> (junction 10) [order 1] : [hasChangedTo(Can_MotorCtrl,0)]
    (junction 7) -> (junction 14) [order 2]
    (junction 10) -> (junction 12) : {StartFlag = TRUE;}
    (junction 12) -> (junction 14)
    (junction 14) -> (junction 17)
    (junction 17) -> (junction 19) [order 1] : /*延时50ms更新接口命令，避免Hall计数错误*/
        | [TRUE == StartFlag]
    (junction 17) -> (junction 28) [order 2] : {Command = Can_MotorCtrl;}
    (junction 19) -> (junction 21)
    (junction 21) -> (junction 31) [order 1] : [CAL_MotorStopTime_50ms > WaitTimer]
    (junction 21) -> (junction 35) [order 2] : {StartFlag = FALSE;
        | WaitTimer = 0;
        | Command = Can_MotorCtrl;}
    (junction 31) -> (junction 33) : {WaitTimer ++;}
    (junction 35) -> (junction 28)
    (junction 33) -> (junction 35)
    (junction 28) -> (junction 39)
  (default) -> Height
  data: Can_MotorCtrl input uint8; StartFlag local uint8; TRUE parameter; WaitTimer local uint8; CAL_MotorStopTime_50ms parameter; Command output uint8; FALSE parameter

== stateflow chart Appl_DrMotorAdjust_CtrlModel/LogicCtrl/LocalAdjustCtrl/FourMotorPriority/FrontDelay ==
  state Height
    (default) -> (junction 7)
    Height -> (junction 7)
    (junction 7) -> (junction 10) [order 1] : [hasChangedTo(Can_MotorCtrl,0)]
    (junction 7) -> (junction 14) [order 2]
    (junction 10) -> (junction 12) : {StartFlag = TRUE;}
    (junction 12) -> (junction 14)
    (junction 14) -> (junction 17)
    (junction 17) -> (junction 19) [order 1] : /*延时50ms更新接口命令，避免Hall计数错误*/
        | [TRUE == StartFlag]
    (junction 17) -> (junction 28) [order 2] : {Command = Can_MotorCtrl;}
    (junction 19) -> (junction 21)
    (junction 21) -> (junction 31) [order 1] : [CAL_MotorStopTime_50ms > WaitTimer]
    (junction 21) -> (junction 35) [order 2] : {StartFlag = FALSE;
        | WaitTimer = 0;
        | Command = Can_MotorCtrl;}
    (junction 31) -> (junction 33) : {WaitTimer ++;}
    (junction 35) -> (junction 28)
    (junction 33) -> (junction 35)
    (junction 28) -> (junction 39)
  (default) -> Height
  data: Can_MotorCtrl input uint8; StartFlag local uint8; TRUE parameter; WaitTimer local uint8; CAL_MotorStopTime_50ms parameter; Command output uint8; FALSE parameter
